simulink model "main"  (R2025b)
settings: Solver=FixedStepDiscrete  StartTime=0.0  StopTime=Inf  RelTol=1e-3  EnableMultiTasking=on
PreLoadFcn:
  | RTWConfigurationCB('preloadfcn', bdroot);
model workspace (MAT data in the model file):
  fault_count = 0
  fz_values = [0 50 100 150 200 250 300 350 400 450 500 550 ... (43 elements, 1x43)]
  k_opt_lut = [0 0 0 0 0 0 0 0 0 0 0 0 ... (4386 elements, 51x2x43)]
  mu_opt_lut = [0 0 0 0 0 0 0 0 0 0 0 0 ... (4386 elements, 51x2x43)]
undefined symbols (not defined in the file or in its folder): bit, Call, Function, ocv_lut, slope_lut, soc_lut
libraries: c2837xDlib x34, c280xlib x20, canmsglib x18, c2802xlib x12, simulink x9, slpidlib x3
(part 4 of 5)

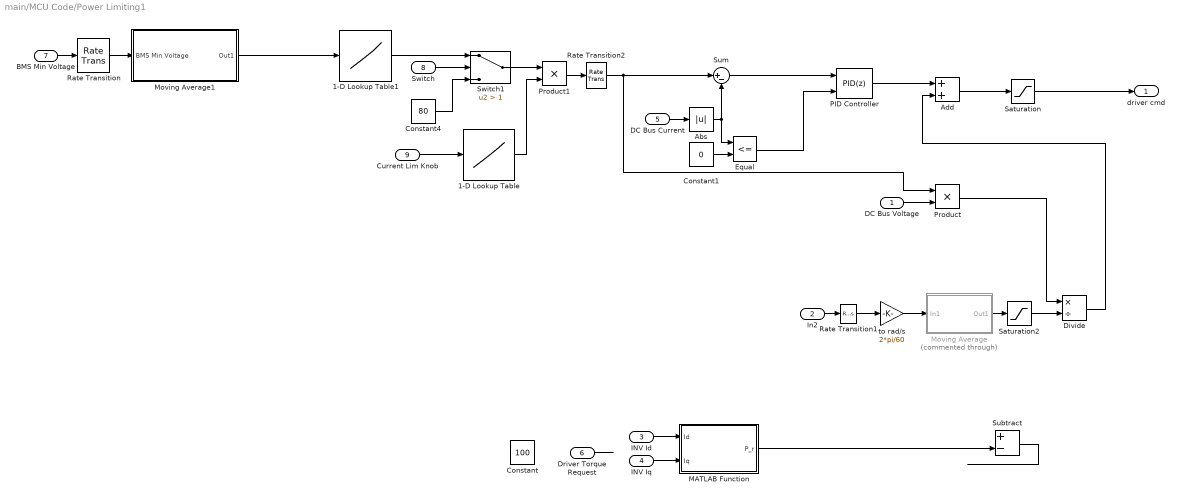
== system main/MCU Code/Power Limiting1 ==
  DC Bus Voltage : Inport
  In2 : Inport  Port=2
  INV Id : Inport  Port=3
  INV Iq : Inport  Port=4
  DC Bus Current : Inport  Port=5
  Driver Torque Request : Inport  Port=6
  BMS Min Voltage : Inport  Port=7
  Switch : Inport  Port=8
  Current Lim Knob : Inport  Port=9
  1-D Lookup Table : Lookup_n-D  NumberOfTableDimensions=1  BreakpointsForDimension1=[1 10]  Table=[0.1 1]  ExtrapMethod=Clip  UseLastTableValue=on  InternalRulePriority=Speed  RndMeth=Simplest
  1-D Lookup Table1 : Lookup_n-D  NumberOfTableDimensions=1  BreakpointsForDimension1=[3.4 4]  Table=[40 80]  ExtrapMethod=Clip  UseLastTableValue=on  InternalRulePriority=Speed  RndMeth=Simplest
  Abs : Abs  SaturateOnIntegerOverflow=off
  Add : Sum
  Constant : Constant  Value=100
  Constant1 : Constant  Value=0
  Constant4 : Constant  Value=80
  Divide : Product  Inputs=*/
  Equal : RelationalOperator  Operator=<=  OutDataTypeStr=boolean  RndMeth=Simplest  InputSameDT=off
  MATLAB Function : MATLAB Function  TreatAsAtomicUnit=on
  Moving Average : Subsystem  Commented=through
  Moving Average1 : Subsystem
  PID Controller : slpidlib/PID Controller  Controller=PID  Form=Parallel  TimeDomain=Discrete-time  UseExternalTs=off  SampleTime=-1  IntegratorMethod=Forward Euler  FilterMethod=Forward Euler  ControllerParametersSource=internal  P=0.45  I=10.8  UseKiTs=off  D=0  UseExternalDerivativeSource=off  N=100  UseFilter=on  TunerSelectOption=Transfer Function Based (PID Tuner App)  InitialConditionSource=internal  InitialConditionForIntegrator=0  InitialConditionForFilter=0  DifferentiatorICPrevScaledInput=0  ExternalReset=level  TrackingMode=off  Kt=1  LimitOutput=on  SatLimitsSource=internal  UpperSaturationLimit=inf  LowerSaturationLimit=-1000  LinearizeAsGain=off  AntiWindupMode=clamping  Kb=1  LimitIntegrator=on  UpperIntegratorSaturationLimit=0  LowerIntegratorSaturationLimit=-1000  POutMin=[]  POutMax=[]  IOutMin=[]  IOutMax=[]  DOutMin=[]  DOutMax=[]  NOutMin=[]  NOutMax=[]  SumOutMin=[]  SumOutMax=[]  SaturationOutMin=[]  SaturationOutMax=[]  PParamMin=[]  PParamMax=[]  IParamMin=[]  IParamMax=[]  DParamMin=[]  DParamMax=[]  NParamMin=[]  NParamMax=[]  KbParamMin=[]  KbParamMax=[]  KtParamMin=[]  KtParamMax=[]  KbOutMin=[]  KbOutMax=[]  KtOutMin=[]  KtOutMax=[]  IntegratorOutMin=[]  IntegratorOutMax=[]  FilterOutMin=[]  FilterOutMax=[]  SumI1OutMin=[]  SumI1OutMax=[]  SumI2OutMin=[]  SumI2OutMax=[]  SumI3OutMin=[]  SumI3OutMax=[]  SumI4OutMin=[]  SumI4OutMax=[]  SumDOutMin=[]  SumDOutMax=[]  DifferentiatorOutMin=[]  DifferentiatorOutMax=[]  FilterDiffOutCoefMin=[]  FilterDiffOutCoefMax=[]  ReciprocalOutMin=[]  ReciprocalOutMax=[]  SumDenOutMin=[]  SumDenOutMax=[]  SumNumOutMin=[]  SumNumOutMax=[]  DivideOutMin=[]  DivideOutMax=[]  UdiffTsProdOutMin=[]  UdiffTsProdOutMax=[]  NTsProdOutMin=[]  NTsProdOutMax=[]  UintegralTsProdOutMin=[]  UintegralTsProdOutMax=[]  UngainTsProdOutMin=[]  UngainTsProdOutMax=[]  ClampingZeroOutDataTypeStr=Inherit: Inherit via back propagation  ClampingZeroOutMin=[]  ClampingZeroOutMax=[]  FilterDenConstantOutDataTypeStr=Inherit: Inherit via back propagation  FilterDenConstantOutMin=[]  FilterDenConstantOutMax=[]  PCopyOutDataTypeStr=Inherit: Inherit via back propagation  PCopyOutMin=[]  PCopyOutMax=[]  NCopyOutDataTypeStr=Inherit: Inherit via back propagation  NCopyOutMin=[]  NCopyOutMax=[]  IntegratorContinuousStateAttributes=''  IntegratorStateMustResolveToSignalObject=off  IntegratorRTWStateStorageClass=Auto  FilterContinuousStateAttributes=''  FilterStateMustResolveToSignalObject=off  FilterRTWStateStorageClass=Auto  ParallelPVariant=InternalParameters  IdealPVariant=Disabled  IVariant=InternalParameters  DVariant=InternalParameters  IntegratorVariant=Discrete  SatVariant=Enabled  AWVariant=DiscClampingParallel  PCopyVariant=Disabled  TRVariant=Disabled  FdbkBlocksVariant=Forward  IdealPFdbkVariant=Disabled  SatFdbkVariant=Disabled  DerivativeFilterVariant=ForwardEulerFilter  NVariant=InternalParameters  NCopyVariant=Disabled  FilterICVariant=InternalICsFilter  IntegratorICVariant=InternalICs  ExternalResetVariant=ExternalReset  TRSumVariant=Passthrough  SumFdbkVariant=Disabled  SumVariant=Sum_PID  TsampFilterVariant=InternalTs  TsampNgainVariant=Passthrough  TsampIntegralVariant=Disabled_SignalSpec  ExternalSaturationOutDataTypeStr=Inherit: Same as second input  DerivativeSourceVariant=ErrorSignal  PreIntVariant=InternalPreInt
  Product : Product
  Product1 : Product
  Rate Transition : RateTransition  InitialCondition=1/5
  Rate Transition1 : RateTransition  OutPortSampleTime=0.001
  Rate Transition2 : RateTransition  OutPortSampleTime=0.001
  Saturation : Saturate  UpperLimit=inf  LowerLimit=0
  Saturation2 : Saturate  UpperLimit=inf  LowerLimit=1
  Subtract : Sum  Inputs=+-
  Sum : Sum  Inputs=|+-
  Switch1 : Switch  Criteria=u2 > Threshold  Threshold=1  SaturateOnIntegerOverflow=off  InputSameDT=off
  to rad/s : Gain  Gain=2*pi/60
  driver cmd : Outport
  wires:
  to rad/s/1 -> Moving Average/1(In1)
  Moving Average/1(Out1) -> Saturation2/1
  Saturation2/1 -> Divide/2
  Product/1 -> Divide/1
  DC Bus Voltage/1 -> Product/2
  In2/1 -> Rate Transition1/1
  INV Id/1 -> MATLAB Function/1(Id)
  INV Iq/1 -> MATLAB Function/2(Iq)
  MATLAB Function/1(P_r) -> Subtract/2
  Subtract/1 -> ?
  DC Bus Current/1 -> Abs/1
  Sum/1 -> PID Controller/1
  PID Controller/1 -> Add/1
  Driver Torque Request/1 -> ?
  Add/1 -> Saturation/1
  Abs/1 -> Sum/2, Equal/1
  Equal/1 -> PID Controller/2
  Product1/1 -> Rate Transition2/1
  Saturation/1 -> driver cmd/1
  Divide/1 -> Add/2
  Constant1/1 -> Equal/2
  BMS Min Voltage/1 -> Rate Transition/1
  Rate Transition/1 -> Moving Average1/1(BMS Min Voltage)
  Constant4/1 -> Switch1/3
  1-D Lookup Table1/1 -> Switch1/1
  Moving Average1/1(Out1) -> 1-D Lookup Table1/1
  Current Lim Knob/1 -> 1-D Lookup Table/1
  Switch1/1 -> Product1/1
  Switch/1 -> Switch1/2
  1-D Lookup Table/1 -> Product1/2
  Rate Transition2/1 -> Product/1, Sum/1
  Rate Transition1/1 -> to rad/s/1

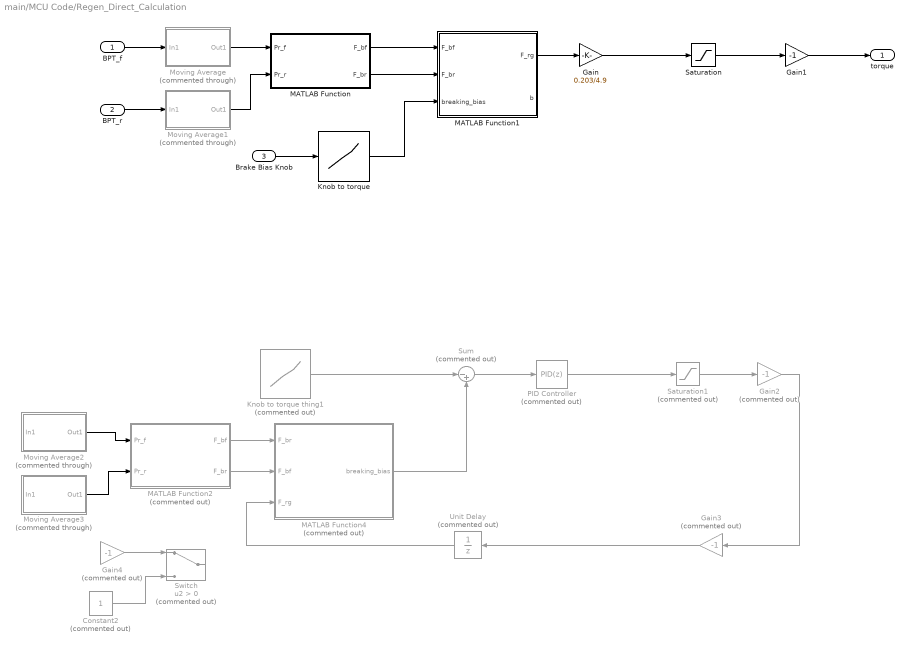
== system main/MCU Code/Regen_Direct_Calculation ==
  BPT_f : Inport
  BPT_r : Inport  Port=2
  Brake Bias Knob : Inport  Port=3
  Constant2 : Constant  Commented=on
  Gain : Gain  Gain=0.203/4.9
  Gain1 : Gain  Gain=-1
  Gain2 : Gain  Commented=on  Gain=-1
  Gain3 : Gain  Commented=on  Gain=-1
  Gain4 : Gain  Commented=on  Gain=-1
  Knob to torque : Lookup_n-D  NumberOfTableDimensions=1  BreakpointsForDimension1=[1 10]  Table=[0 1]  InternalRulePriority=Speed  RndMeth=Simplest
  Knob to torque thing1 : Lookup_n-D  Commented=on  NumberOfTableDimensions=1  BreakpointsForDimension1=[1 10]  Table=[0 1]  InternalRulePriority=Speed  RndMeth=Simplest
  MATLAB Function : MATLAB Function  TreatAsAtomicUnit=on
  MATLAB Function1 : MATLAB Function  TreatAsAtomicUnit=on
  MATLAB Function2 : MATLAB Function  Commented=on  TreatAsAtomicUnit=on
  MATLAB Function4 : MATLAB Function  Commented=on  TreatAsAtomicUnit=on
  Moving Average : Subsystem  Commented=through
  Moving Average1 : Subsystem  Commented=through
  Moving Average2 : Subsystem  Commented=through
  Moving Average3 : Subsystem  Commented=through
  PID Controller : slpidlib/PID Controller  Commented=on  Controller=PID  Form=Parallel  TimeDomain=Discrete-time  UseExternalTs=off  SampleTime=-1  IntegratorMethod=Forward Euler  FilterMethod=Forward Euler  ControllerParametersSource=internal  P=30  I=5000  UseKiTs=off  D=0  UseExternalDerivativeSource=off  N=100  UseFilter=on  TunerSelectOption=Transfer Function Based (PID Tuner App)  InitialConditionSource=internal  InitialConditionForIntegrator=0  InitialConditionForFilter=0  DifferentiatorICPrevScaledInput=0  ExternalReset=none  TrackingMode=off  Kt=1  LimitOutput=on  SatLimitsSource=internal  UpperSaturationLimit=inf  LowerSaturationLimit=-inf  LinearizeAsGain=on  AntiWindupMode=clamping  Kb=1  LimitIntegrator=off  UpperIntegratorSaturationLimit=inf  LowerIntegratorSaturationLimit=-inf  POutMin=[]  POutMax=[]  IOutMin=[]  IOutMax=[]  DOutMin=[]  DOutMax=[]  NOutMin=[]  NOutMax=[]  SumOutMin=[]  SumOutMax=[]  SaturationOutMin=[]  SaturationOutMax=[]  PParamMin=[]  PParamMax=[]  IParamMin=[]  IParamMax=[]  DParamMin=[]  DParamMax=[]  NParamMin=[]  NParamMax=[]  KbParamMin=[]  KbParamMax=[]  KtParamMin=[]  KtParamMax=[]  KbOutMin=[]  KbOutMax=[]  KtOutMin=[]  KtOutMax=[]  IntegratorOutMin=[]  IntegratorOutMax=[]  FilterOutMin=[]  FilterOutMax=[]  SumI1OutMin=[]  SumI1OutMax=[]  SumI2OutMin=[]  SumI2OutMax=[]  SumI3OutMin=[]  SumI3OutMax=[]  SumI4OutMin=[]  SumI4OutMax=[]  SumDOutMin=[]  SumDOutMax=[]  DifferentiatorOutMin=[]  DifferentiatorOutMax=[]  FilterDiffOutCoefMin=[]  FilterDiffOutCoefMax=[]  ReciprocalOutMin=[]  ReciprocalOutMax=[]  SumDenOutMin=[]  SumDenOutMax=[]  SumNumOutMin=[]  SumNumOutMax=[]  DivideOutMin=[]  DivideOutMax=[]  UdiffTsProdOutMin=[]  UdiffTsProdOutMax=[]  NTsProdOutMin=[]  NTsProdOutMax=[]  UintegralTsProdOutMin=[]  UintegralTsProdOutMax=[]  UngainTsProdOutMin=[]  UngainTsProdOutMax=[]  ClampingZeroOutDataTypeStr=Inherit: Inherit via back propagation  ClampingZeroOutMin=[]  ClampingZeroOutMax=[]  FilterDenConstantOutDataTypeStr=Inherit: Inherit via back propagation  FilterDenConstantOutMin=[]  FilterDenConstantOutMax=[]  PCopyOutDataTypeStr=Inherit: Inherit via back propagation  PCopyOutMin=[]  PCopyOutMax=[]  NCopyOutDataTypeStr=Inherit: Inherit via back propagation  NCopyOutMin=[]  NCopyOutMax=[]  IntegratorContinuousStateAttributes=''  IntegratorStateMustResolveToSignalObject=off  IntegratorRTWStateStorageClass=Auto  FilterContinuousStateAttributes=''  FilterStateMustResolveToSignalObject=off  FilterRTWStateStorageClass=Auto  ParallelPVariant=InternalParameters  IdealPVariant=Disabled  IVariant=InternalParameters  DVariant=InternalParameters  IntegratorVariant=Discrete  SatVariant=Enabled  AWVariant=DiscClampingParallel  PCopyVariant=Disabled  TRVariant=Disabled  FdbkBlocksVariant=Forward  IdealPFdbkVariant=Disabled  SatFdbkVariant=Disabled  DerivativeFilterVariant=ForwardEulerFilter  NVariant=InternalParameters  NCopyVariant=Disabled  FilterICVariant=InternalICsFilter  IntegratorICVariant=InternalICs  ExternalResetVariant=Disabled  TRSumVariant=Passthrough  SumFdbkVariant=Disabled  SumVariant=Sum_PID  TsampFilterVariant=InternalTs  TsampNgainVariant=Passthrough  TsampIntegralVariant=Disabled_SignalSpec  ExternalSaturationOutDataTypeStr=Inherit: Same as second input  DerivativeSourceVariant=ErrorSignal  PreIntVariant=InternalPreInt
  Saturation : Saturate  UpperLimit=100  LowerLimit=0
  Saturation1 : Saturate  Commented=on  UpperLimit=100  LowerLimit=0
  Sum : Sum  Commented=on  Inputs=|-+
  Switch : Switch  Commented=on  Criteria=u2 > Threshold  SaturateOnIntegerOverflow=off  InputSameDT=off
  Unit Delay : UnitDelay  Commented=on  SampleTime=-1  HasFrameUpgradeWarning=on
  torque : Outport
  wires:
  Gain1/1 -> torque/1
  Gain/1 -> Saturation/1
  Brake Bias Knob/1 -> Knob to torque/1
  BPT_f/1 -> Moving Average/1(In1)
  BPT_r/1 -> Moving Average1/1(In1)
  MATLAB Function/1(F_bf) -> MATLAB Function1/1(F_bf)
  MATLAB Function/2(F_br) -> MATLAB Function1/2(F_br)
  MATLAB Function1/1(F_rg) -> Gain/1
  Moving Average/1(Out1) -> MATLAB Function/1(Pr_f)
  Moving Average1/1(Out1) -> MATLAB Function/2(Pr_r)
  Knob to torque/1 -> MATLAB Function1/3(breaking_bias)
  ? -> Moving Average2/1(In1)
  Moving Average2/1(Out1) -> MATLAB Function2/1(Pr_f)
  Sum/1 -> PID Controller/1
  PID Controller/1 -> Saturation1/1
  MATLAB Function2/1(F_bf) -> MATLAB Function4/1(F_br)
  ? -> Moving Average3/1(In1)
  Saturation1/1 -> Gain2/1
  MATLAB Function4/1(breaking_bias) -> Sum/2
  Knob to torque thing1/1 -> Sum/1
  MATLAB Function2/2(F_br) -> MATLAB Function4/2(F_bf)
  Unit Delay/1 -> MATLAB Function4/3(F_rg)
  Moving Average3/1(Out1) -> MATLAB Function2/2(Pr_r)
  Gain3/1 -> Unit Delay/1
  Gain4/1 -> Switch/1
  ? -> Gain4/1
  Constant2/1 -> Switch/3
  ? -> Switch/2
  Saturation/1 -> Gain1/1
  Gain2/1 -> Gain3/1

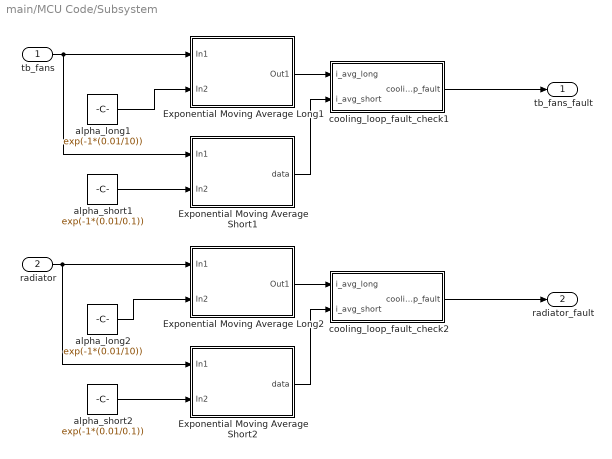
== system main/MCU Code/Subsystem ==
  tb_fans : Inport
  radiator : Inport  Port=2
  Exponential Moving Average Long1 : Subsystem
  Exponential Moving Average Long2 : Subsystem
  Exponential Moving Average Short1 : Subsystem
  Exponential Moving Average Short2 : Subsystem
  alpha_long1 : Constant  Value=exp(-1*(0.01/10))  VectorParams1D=off
  alpha_long2 : Constant  Value=exp(-1*(0.01/10))
  alpha_short1 : Constant  Value=exp(-1*(0.01/0.1))
  alpha_short2 : Constant  Value=exp(-1*(0.01/0.1))
  cooling_loop_fault_check1 : MATLAB Function  TreatAsAtomicUnit=on
  cooling_loop_fault_check2 : MATLAB Function  TreatAsAtomicUnit=on
  tb_fans_fault : Outport
  radiator_fault : Outport  Port=2
  wires:
  alpha_long1/1 -> Exponential Moving Average Long1/2(In2)
  Exponential Moving Average Short2/1(data) -> cooling_loop_fault_check2/2(i_avg_short)
  Exponential Moving Average Short1/1(data) -> cooling_loop_fault_check1/2(i_avg_short)
  Exponential Moving Average Long1/1(Out1) -> cooling_loop_fault_check1/1(i_avg_long)
  Exponential Moving Average Long2/1(Out1) -> cooling_loop_fault_check2/1(i_avg_long)
  alpha_long2/1 -> Exponential Moving Average Long2/2(In2)
  alpha_short1/1 -> Exponential Moving Average Short1/2(In2)
  alpha_short2/1 -> Exponential Moving Average Short2/2(In2)
  cooling_loop_fault_check1/1(cooling_loop_fault) -> tb_fans_fault/1
  cooling_loop_fault_check2/1(cooling_loop_fault) -> radiator_fault/1
  tb_fans/1 -> Exponential Moving Average Short1/1(In1), Exponential Moving Average Long1/1(In1)
  radiator/1 -> Exponential Moving Average Short2/1(In1), Exponential Moving Average Long2/1(In1)

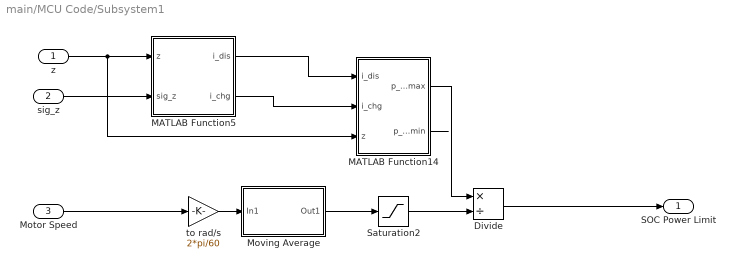
== system main/MCU Code/Subsystem1 ==
  z : Inport
  sig_z : Inport  Port=2
  Motor Speed : Inport  Port=3
  Divide : Product  Inputs=*/
  MATLAB Function14 : MATLAB Function  TreatAsAtomicUnit=on
  MATLAB Function5 : MATLAB Function  TreatAsAtomicUnit=on
  Moving Average : Subsystem
  Saturation2 : Saturate  UpperLimit=inf  LowerLimit=1
  to rad/s : Gain  Gain=2*pi/60
  SOC Power Limit : Outport
  wires:
  to rad/s/1 -> Moving Average/1(In1)
  MATLAB Function5/2(i_chg) -> MATLAB Function14/2(i_chg)
  Saturation2/1 -> Divide/2
  Motor Speed/1 -> to rad/s/1
  Moving Average/1(Out1) -> Saturation2/1
  MATLAB Function14/1(p_dis_max) -> Divide/1
  z/1 -> MATLAB Function5/1(z), MATLAB Function14/3(z)
  MATLAB Function5/1(i_dis) -> MATLAB Function14/1(i_dis)
  Divide/1 -> SOC Power Limit/1
  MATLAB Function14/2(p_chg_min) -> ?
  sig_z/1 -> MATLAB Function5/2(sig_z)

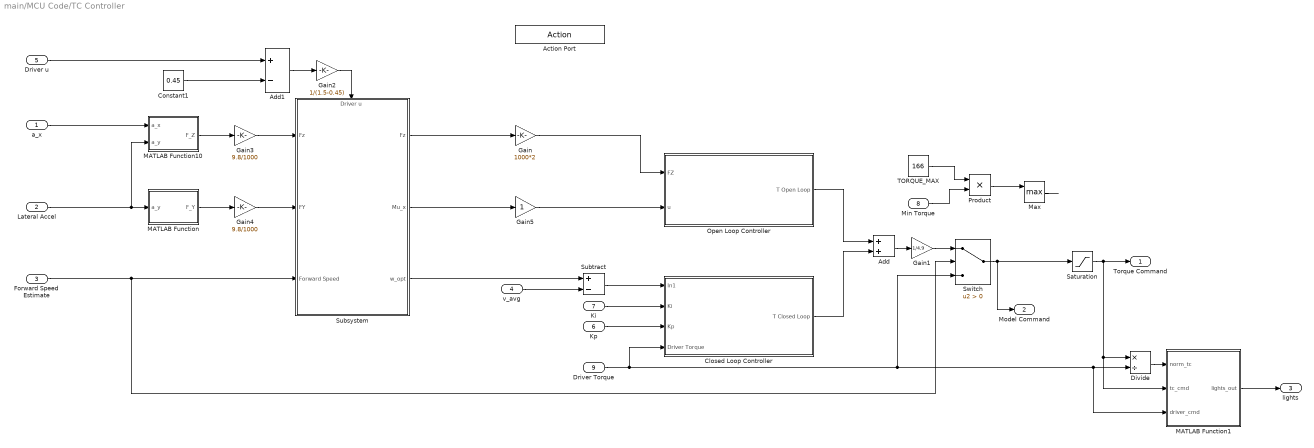
== system main/MCU Code/TC Controller ==
  a_x : Inport
  Lateral Accel : Inport  Port=2
  Forward Speed Estimate : Inport  Port=3
  v_avg : Inport  Port=4
  Driver u : Inport  Port=5
  Kp : Inport  Port=6
  Ki : Inport  Port=7
  Min Torque : Inport  Port=8
  Driver Torque : Inport  Port=9
  Action Port : ActionPort  ActionPortLabel=|
      | if(u1 == 1 | u1 == 3
      | )
  Add : Sum
  Add1 : Sum  Inputs=+-
  Closed Loop Controller : Subsystem
  Constant1 : Constant  Value=0.45
  Divide : Product  Inputs=*/
  Gain : Gain  Gain=1000*2
  Gain1 : Gain  Gain=1/4.9
  Gain2 : Gain  Gain=1/(1.5-0.45)
  Gain3 : Gain  Gain=9.8/1000
  Gain4 : Gain  Gain=9.8/1000
  Gain5 : Gain
  MATLAB Function : MATLAB Function  TreatAsAtomicUnit=on
  MATLAB Function1 : MATLAB Function  TreatAsAtomicUnit=on
  MATLAB Function10 : MATLAB Function  TreatAsAtomicUnit=on
  Max : MinMax  Function=max  Inputs=2
  Open Loop Controller : Subsystem
  Product : Product
  Saturation : Saturate  UpperLimit=166  LowerLimit=0
  Subsystem : Subsystem
      settings: PortSchema="{\"entries\":[{\"content\":{\"sides\":[{\"content\":{\"connectorIds\":[\"In1\",\"In2\",\"In3\"]},\"type\":\"ConnectorPlacement.EquallySpacedRectSide\",\"uuid\":\"52cb1509-e05e-4bae-af08-b3cbe80ce8d7\"},{\"content\":{\"connectorIds\":[\"Out1\",\"Out2\",\"Out3\"],\"side\":\"RIGHT\"},\"type\":\"ConnectorPlacement.EquallySpacedRectSide\",\"uuid\":\"5c1b6c4d-f36b-4262-971d-310d950de965\"},{\"content\":{\"connectorIds\":[\"In4\"],\"side\":\"TOP\"},\"type\":\"ConnectorPlacement.EquallySpacedRectSide\",\"uuid\":\"90df2961-afb4-4b60-bc78-aaa8af520e7a\"}]},\"type\":\"ConnectorPlacement.EquallySpacedConnector\",\"uuid\":\"073ed346-9857-4a79-b76f-e1da7d32971a\"}],\"packageUris\":[\"http://schema.mathworks.com/mf0/Connector/R2020b\"],\"version\":\"1.0\"}"
  Subtract : Sum  Inputs=+-
  Switch : Switch  Criteria=u2 > Threshold  SaturateOnIntegerOverflow=off  InputSameDT=off
  TORQUE_MAX : Constant  Value=166
  Torque Command : Outport
  Model Command : Outport  Port=2
  lights : Outport  Port=3
  wires:
  Gain1/1 -> Switch/1
  MATLAB Function10/1(F_Z) -> Gain3/1
  Open Loop Controller/1(T Open Loop) -> Add/1
  Closed Loop Controller/1(T Closed Loop) -> Add/2
  Add/1 -> Gain1/1
  v_avg/1 -> Subtract/2
  Kp/1 -> Closed Loop Controller/3(Kp)
  Forward Speed Estimate/1 -> Subsystem/3(Forward Speed), Switch/2
  Ki/1 -> Closed Loop Controller/2(Ki)
  Switch/1 -> Saturation/1, Model Command/1
  TORQUE_MAX/1 -> Product/1
  Min Torque/1 -> Product/2
  Lateral Accel/1 -> MATLAB Function10/2(a_y), MATLAB Function/1(a_y)
  Driver u/1 -> Add1/1
  Constant1/1 -> Add1/2
  Add1/1 -> Gain2/1
  Gain2/1 -> Subsystem/4(Driver u)
  Subsystem/3(w_opt) -> Subtract/1
  Subsystem/1(Fz) -> Gain/1
  Subsystem/2(Mu_x) -> Gain5/1
  Gain4/1 -> Subsystem/2(FY)
  MATLAB Function/1(F_Y) -> Gain4/1
  Gain3/1 -> Subsystem/1("Fz ")
  a_x/1 -> MATLAB Function10/1(a_x)
  Gain/1 -> Open Loop Controller/1(FZ)
  Gain5/1 -> Open Loop Controller/2(u)
  Subtract/1 -> Closed Loop Controller/1(In1)
  Saturation/1 -> Divide/1, MATLAB Function1/2(tc_cmd), Torque Command/1
  Max/1 -> ?
  Product/1 -> Max/1
  Driver Torque/1 -> Closed Loop Controller/4(Driver Torque), Switch/3, MATLAB Function1/3(driver_cmd), Divide/2
  Divide/1 -> MATLAB Function1/1(norm_tc)
  MATLAB Function1/1(lights_out) -> lights/1

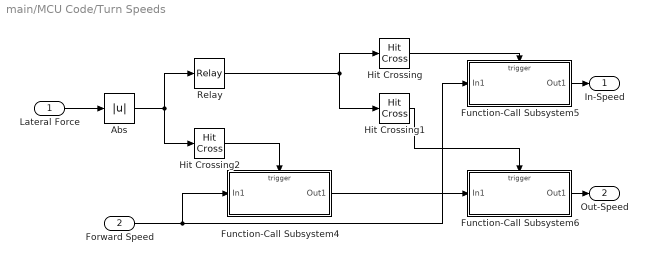
== system main/MCU Code/Turn Speeds ==
  Lateral Force : Inport
  Forward Speed : Inport  Port=2
  Abs : Abs  SaturateOnIntegerOverflow=off
  Function-Call Subsystem4 : Subsystem  TreatAsAtomicUnit=on
  Function-Call Subsystem5 : Subsystem  TreatAsAtomicUnit=on
  Function-Call Subsystem6 : Subsystem  TreatAsAtomicUnit=on
  Hit Crossing : HitCross  HitCrossingOffset=0.5  HitCrossingDirection=rising  HitCrossingOutputType=Function-Call
  Hit Crossing1 : HitCross  HitCrossingOffset=0.5  HitCrossingDirection=falling  HitCrossingOutputType=Function-Call
  Hit Crossing2 : HitCross  HitCrossingOffset=1  HitCrossingOutputType=Function-Call
  Relay : Relay  OnSwitchValue=1  OffSwitchValue=0.5
  In-Speed : Outport
  Out-Speed : Outport  Port=2
  wires:
  Forward Speed/1 -> Function-Call Subsystem4/1(In1), Function-Call Subsystem5/1(In1)
  Hit Crossing2/1 -> Function-Call Subsystem4/Trigger
  Function-Call Subsystem4/1(Out1) -> Function-Call Subsystem6/1(In1)
  Relay/1 -> Hit Crossing1/1, Hit Crossing/1
  Hit Crossing1/1 -> Function-Call Subsystem6/Trigger
  Hit Crossing/1 -> Function-Call Subsystem5/Trigger
  Function-Call Subsystem5/1(Out1) -> In-Speed/1
  Lateral Force/1 -> Abs/1
  Function-Call Subsystem6/1(Out1) -> Out-Speed/1
  Abs/1 -> Relay/1, Hit Crossing2/1

== system main/Subsystem/Subsystem3 ==
  In1 : Inport
  In2 : Inport  Port=2
  Forward Speed Estimate : Inport  Port=3
  In4 : Inport  Port=4
  Enable : EnablePort

== system main/MCU Code/Kalman Filter/Kalman1 ==
  Accel : Inport
  Speed F : Inport  Port=2
  Accel update : Inport  Port=3
  Velocity Update : Inport  Port=4
  Time : Inport  Port=5
  MATLAB System : MATLABSystem  System=Kalman_Filter_Mod  qgain=1  SimulateUsing=Code generation
      mask Type: Kalman_Filter_Mod
  Forward Speed : Outport
  Accel Estimate : Outport  Port=2
  Error Covariance : Outport  Port=3
  wires:
  Speed F/1 -> MATLAB System/2
  Accel/1 -> MATLAB System/1
  MATLAB System/1 -> Forward Speed/1
  Accel update/1 -> MATLAB System/3
  Velocity Update/1 -> MATLAB System/4
  Time/1 -> MATLAB System/5
  MATLAB System/2 -> Accel Estimate/1
  MATLAB System/3 -> Error Covariance/1

== system main/MCU Code/Kalman Filter/Sensor Driver 1 ==
  In1 : Inport
  Circumference : Gain  Gain=2*pi*0.203
  Gain : Gain  Gain=3.6
  Inverse Teeth : Gain  Gain=1/21
  " " : Outport
  wires:
  In1/1 -> Gain/1
  Gain/1 -> Circumference/1
  Circumference/1 -> Inverse Teeth/1
  Inverse Teeth/1 -> " "/1

== system main/MCU Code/Kalman Filter/Sensor Driver 2 ==
  In1 : Inport
  Circumference : Gain  Gain=2*pi*0.203
  Gain : Gain  Gain=3.6
  Inverse Teeth : Gain  Gain=1/21
  " " : Outport
  wires:
  Circumference/1 -> Inverse Teeth/1
  Inverse Teeth/1 -> " "/1
  In1/1 -> Gain/1
  Gain/1 -> Circumference/1

== system main/MCU Code/Kalman Filter/Sensor Driver 3 ==
  In1 : Inport
  Circumference : Gain  Gain=2*pi*0.203
  Gain : Gain  Gain=3.6
  Inverse Teeth : Gain  Gain=1/21
  RL : Outport
  wires:
  Circumference/1 -> Inverse Teeth/1
  Inverse Teeth/1 -> RL/1
  In1/1 -> Gain/1
  Gain/1 -> Circumference/1

== system main/MCU Code/Kalman Filter/Sensor Driver 4 ==
  In1 : Inport
  Circumference : Gain  Gain=2*pi*0.203
  Gain : Gain  Gain=3.6
  Inverse Teeth : Gain  Gain=1/21
  RR : Outport
  wires:
  Circumference/1 -> Inverse Teeth/1
  Inverse Teeth/1 -> RR/1
  In1/1 -> Gain/1
  Gain/1 -> Circumference/1

== system main/MCU Code/Kalman Filter/Slip Ratio Calculation1 ==
  RR : Inport
  Forward Speed : Inport  Port=2
  MATLAB Function : MATLAB Function  TreatAsAtomicUnit=on
  Slip Ratio : Outport
  wires:
  Forward Speed/1 -> MATLAB Function/1(fwd_speed)
  RR/1 -> MATLAB Function/2(v_rear)
  MATLAB Function/1(y) -> Slip Ratio/1

== system main/MCU Code/Power Limiting/Moving Average ==
  In1 : Inport
  Product1 : Product  Inputs=*/
  Saturation : Saturate  UpperLimit=inf  LowerLimit=1
  Sum of Elements : Sum  Inputs=+
  Tapped Delay : simulink/Discrete/Tapped Delay  vinit=0.0  samptime=-1  NumDelays=10  DelayOrder=Oldest  includeCurrent=on
  Width : Width
  Out1 : Outport
  wires:
  Tapped Delay/1 -> Width/1, Sum of Elements/1
  Sum of Elements/1 -> Product1/1
  Product1/1 -> Out1/1
  In1/1 -> Tapped Delay/1
  Width/1 -> Saturation/1
  Saturation/1 -> Product1/2

== system main/MCU Code/Power Limiting1/Moving Average ==
  In1 : Inport
  Product1 : Product  Inputs=*/
  Saturation : Saturate  UpperLimit=inf  LowerLimit=1
  Sum of Elements : Sum  Inputs=+
  Tapped Delay : simulink/Discrete/Tapped Delay  vinit=0.0  samptime=-1  NumDelays=10  DelayOrder=Oldest  includeCurrent=on
  Width : Width
  Out1 : Outport
  wires:
  Tapped Delay/1 -> Width/1, Sum of Elements/1
  Sum of Elements/1 -> Product1/1
  Product1/1 -> Out1/1
  In1/1 -> Tapped Delay/1
  Width/1 -> Saturation/1
  Saturation/1 -> Product1/2

== system main/MCU Code/Power Limiting1/Moving Average1 ==
  BMS Min Voltage : Inport
  Product1 : Product  Inputs=*/
  Saturation : Saturate  UpperLimit=inf  LowerLimit=1
  Sum of Elements : Sum  Inputs=+
  Tapped Delay : simulink/Discrete/Tapped Delay  vinit=0.0  samptime=-1  NumDelays=50  DelayOrder=Oldest  includeCurrent=on
  Width : Width
  Out1 : Outport
  wires:
  Tapped Delay/1 -> Width/1, Sum of Elements/1
  Sum of Elements/1 -> Product1/1
  Product1/1 -> Out1/1
  BMS Min Voltage/1 -> Tapped Delay/1
  Width/1 -> Saturation/1
  Saturation/1 -> Product1/2

== system main/MCU Code/Regen_Direct_Calculation/Moving Average ==
  In1 : Inport
  Product1 : Product  Inputs=*/
  Saturation : Saturate  UpperLimit=inf  LowerLimit=1
  Sum of Elements : Sum  Inputs=+
  Tapped Delay : simulink/Discrete/Tapped Delay  vinit=0.0  samptime=-1  NumDelays=10  DelayOrder=Oldest  includeCurrent=on
  Width : Width
  Out1 : Outport
  wires:
  Tapped Delay/1 -> Width/1, Sum of Elements/1
  Sum of Elements/1 -> Product1/1
  Product1/1 -> Out1/1
  In1/1 -> Tapped Delay/1
  Width/1 -> Saturation/1
  Saturation/1 -> Product1/2

== system main/MCU Code/Regen_Direct_Calculation/Moving Average1 ==
  In1 : Inport
  Product1 : Product  Inputs=*/
  Saturation : Saturate  UpperLimit=inf  LowerLimit=1
  Sum of Elements : Sum  Inputs=+
  Tapped Delay : simulink/Discrete/Tapped Delay  vinit=0.0  samptime=-1  NumDelays=10  DelayOrder=Oldest  includeCurrent=on
  Width : Width
  Out1 : Outport
  wires:
  Tapped Delay/1 -> Width/1, Sum of Elements/1
  Sum of Elements/1 -> Product1/1
  Product1/1 -> Out1/1
  In1/1 -> Tapped Delay/1
  Width/1 -> Saturation/1
  Saturation/1 -> Product1/2

== system main/MCU Code/Regen_Direct_Calculation/Moving Average2 ==
  In1 : Inport
  Product1 : Product  Inputs=*/
  Saturation : Saturate  UpperLimit=inf  LowerLimit=1
  Sum of Elements : Sum  Inputs=+
  Tapped Delay : simulink/Discrete/Tapped Delay  vinit=0.0  samptime=-1  NumDelays=10  DelayOrder=Oldest  includeCurrent=on
  Width : Width
  Out1 : Outport
  wires:
  Tapped Delay/1 -> Width/1, Sum of Elements/1
  Sum of Elements/1 -> Product1/1
  Product1/1 -> Out1/1
  In1/1 -> Tapped Delay/1
  Width/1 -> Saturation/1
  Saturation/1 -> Product1/2

== system main/MCU Code/Regen_Direct_Calculation/Moving Average3 ==
  In1 : Inport
  Product1 : Product  Inputs=*/
  Saturation : Saturate  UpperLimit=inf  LowerLimit=1
  Sum of Elements : Sum  Inputs=+
  Tapped Delay : simulink/Discrete/Tapped Delay  vinit=0.0  samptime=-1  NumDelays=10  DelayOrder=Oldest  includeCurrent=on
  Width : Width
  Out1 : Outport
  wires:
  Tapped Delay/1 -> Width/1, Sum of Elements/1
  Sum of Elements/1 -> Product1/1
  Product1/1 -> Out1/1
  In1/1 -> Tapped Delay/1
  Width/1 -> Saturation/1
  Saturation/1 -> Product1/2

== system main/MCU Code/Subsystem/Exponential Moving Average Long1 ==
  In1 : Inport
  In2 : Inport  Port=2
  Constant4 : Constant
  Delay One Step : Delay  DelayLength=1
  Product : Product
  Product1 : Product
  Subtract : Sum  Inputs=+-
  Sum : Sum  Inputs=|++
  Out1 : Outport
  wires:
  In2/1 -> Subtract/2, Product1/2
  Product1/1 -> Sum/1
  Subtract/1 -> Product/2
  Sum/1 -> Out1/1, Delay One Step/1
  Constant4/1 -> Subtract/1
  Product/1 -> Sum/2
  Delay One Step/1 -> Product/1
  In1/1 -> Product1/1

== system main/MCU Code/Subsystem/Exponential Moving Average Long2 ==
  In1 : Inport
  In2 : Inport  Port=2
  Constant4 : Constant
  Delay One Step : Delay  DelayLength=1
  Product : Product
  Product1 : Product
  Subtract : Sum  Inputs=+-
  Sum : Sum  Inputs=|++
  Out1 : Outport
  wires:
  In2/1 -> Subtract/2, Product1/2
  Product1/1 -> Sum/1
  Subtract/1 -> Product/2
  Sum/1 -> Out1/1, Delay One Step/1
  Constant4/1 -> Subtract/1
  Product/1 -> Sum/2
  Delay One Step/1 -> Product/1
  In1/1 -> Product1/1

== system main/MCU Code/Subsystem/Exponential Moving Average Short1 ==
  In1 : Inport
  In2 : Inport  Port=2
  Constant4 : Constant
  Delay One Step : Delay  DelayLength=1
  Product : Product
  Product1 : Product
  Subtract : Sum  Inputs=+-
  Sum : Sum  Inputs=|++
  data : Outport
  wires:
  In2/1 -> Subtract/2, Product1/2
  Product1/1 -> Sum/1
  Subtract/1 -> Product/2
  Sum/1 -> data/1, Delay One Step/1
  Constant4/1 -> Subtract/1
  Product/1 -> Sum/2
  Delay One Step/1 -> Product/1
  In1/1 -> Product1/1

== system main/MCU Code/Subsystem/Exponential Moving Average Short2 ==
  In1 : Inport
  In2 : Inport  Port=2
  Constant4 : Constant
  Delay One Step : Delay  DelayLength=1
  Product : Product
  Product1 : Product
  Subtract : Sum  Inputs=+-
  Sum : Sum  Inputs=|++
  data : Outport
  wires:
  In2/1 -> Subtract/2, Product1/2
  Product1/1 -> Sum/1
  Subtract/1 -> Product/2
  Sum/1 -> data/1, Delay One Step/1
  Constant4/1 -> Subtract/1
  Product/1 -> Sum/2
  Delay One Step/1 -> Product/1
  In1/1 -> Product1/1

== system main/MCU Code/Subsystem1/Moving Average ==
  In1 : Inport
  Product1 : Product  Inputs=*/
  Saturation : Saturate  UpperLimit=inf  LowerLimit=1
  Sum of Elements : Sum  Inputs=+
  Tapped Delay : simulink/Discrete/Tapped Delay  vinit=0.0  samptime=-1  NumDelays=10  DelayOrder=Oldest  includeCurrent=on
  Width : Width
  Out1 : Outport
  wires:
  Tapped Delay/1 -> Width/1, Sum of Elements/1
  Sum of Elements/1 -> Product1/1
  Product1/1 -> Out1/1
  In1/1 -> Tapped Delay/1
  Width/1 -> Saturation/1
  Saturation/1 -> Product1/2

== system main/MCU Code/TC Controller/Closed Loop Controller ==
  In1 : Inport
  Ki : Inport  Port=2
  Kp : Inport  Port=3
  Driver Torque : Inport  Port=4
  Constant : Constant  Value=0
  Equal : RelationalOperator  Operator===  OutDataTypeStr=boolean  RndMeth=Simplest  InputSameDT=off
  PID Controller : slpidlib/PID Controller  Controller=PI  Form=Parallel  TimeDomain=Discrete-time  UseExternalTs=off  SampleTime=-1  IntegratorMethod=Forward Euler  FilterMethod=Forward Euler  ControllerParametersSource=external  P=100  I=10  UseKiTs=off  D=0  UseExternalDerivativeSource=off  N=100  UseFilter=on  TunerSelectOption=Transfer Function Based (PID Tuner App)  InitialConditionSource=internal  InitialConditionForIntegrator=0  InitialConditionForFilter=0  DifferentiatorICPrevScaledInput=0  ExternalReset=level  TrackingMode=off  Kt=1  LimitOutput=on  SatLimitsSource=internal  UpperSaturationLimit=166*4.9  LowerSaturationLimit=-166*4.9  LinearizeAsGain=on  AntiWindupMode=clamping  Kb=1  LimitIntegrator=on  UpperIntegratorSaturationLimit=166*4.9  LowerIntegratorSaturationLimit=-166*4.9  POutMin=[]  POutMax=[]  IOutMin=[]  IOutMax=[]  DOutMin=[]  DOutMax=[]  NOutMin=[]  NOutMax=[]  SumOutMin=[]  SumOutMax=[]  SaturationOutMin=[]  SaturationOutMax=[]  PParamMin=[]  PParamMax=[]  IParamMin=[]  IParamMax=[]  DParamMin=[]  DParamMax=[]  NParamMin=[]  NParamMax=[]  KbParamMin=[]  KbParamMax=[]  KtParamMin=[]  KtParamMax=[]  KbOutMin=[]  KbOutMax=[]  KtOutMin=[]  KtOutMax=[]  IntegratorOutMin=[]  IntegratorOutMax=[]  FilterOutMin=[]  FilterOutMax=[]  SumI1OutMin=[]  SumI1OutMax=[]  SumI2OutMin=[]  SumI2OutMax=[]  SumI3OutMin=[]  SumI3OutMax=[]  SumI4OutMin=[]  SumI4OutMax=[]  SumDOutMin=[]  SumDOutMax=[]  DifferentiatorOutMin=[]  DifferentiatorOutMax=[]  FilterDiffOutCoefMin=[]  FilterDiffOutCoefMax=[]  ReciprocalOutMin=[]  ReciprocalOutMax=[]  SumDenOutMin=[]  SumDenOutMax=[]  SumNumOutMin=[]  SumNumOutMax=[]  DivideOutMin=[]  DivideOutMax=[]  UdiffTsProdOutMin=[]  UdiffTsProdOutMax=[]  NTsProdOutMin=[]  NTsProdOutMax=[]  UintegralTsProdOutMin=[]  UintegralTsProdOutMax=[]  UngainTsProdOutMin=[]  UngainTsProdOutMax=[]  ClampingZeroOutDataTypeStr=Inherit: Inherit via back propagation  ClampingZeroOutMin=[]  ClampingZeroOutMax=[]  FilterDenConstantOutDataTypeStr=Inherit: Inherit via back propagation  FilterDenConstantOutMin=[]  FilterDenConstantOutMax=[]  PCopyOutDataTypeStr=Inherit: Inherit via back propagation  PCopyOutMin=[]  PCopyOutMax=[]  NCopyOutDataTypeStr=Inherit: Inherit via back propagation  NCopyOutMin=[]  NCopyOutMax=[]  IntegratorContinuousStateAttributes=''  IntegratorStateMustResolveToSignalObject=off  IntegratorRTWStateStorageClass=Auto  FilterContinuousStateAttributes=''  FilterStateMustResolveToSignalObject=off  FilterRTWStateStorageClass=Auto  ParallelPVariant=ExternalParameters  IdealPVariant=Disabled  IVariant=ExternalParameters  DVariant=Disabled  IntegratorVariant=Discrete  SatVariant=Enabled  AWVariant=DiscClampingParallel  PCopyVariant=Disabled  TRVariant=Disabled  FdbkBlocksVariant=Forward  IdealPFdbkVariant=Disabled  SatFdbkVariant=Disabled  DerivativeFilterVariant=Disabled  NVariant=Disabled  NCopyVariant=Disabled_SignalSpec  FilterICVariant=Disabled  IntegratorICVariant=InternalICs  ExternalResetVariant=ExternalReset  TRSumVariant=Passthrough  SumFdbkVariant=Disabled  SumVariant=Sum_PI  TsampFilterVariant=InternalTs  TsampNgainVariant=Passthrough  TsampIntegralVariant=Disabled_SignalSpec  ExternalSaturationOutDataTypeStr=Inherit: Same as second input  DerivativeSourceVariant=Disabled  PreIntVariant=InternalPreInt
  T Closed Loop : Outport
  wires:
  In1/1 -> PID Controller/1
  PID Controller/1 -> T Closed Loop/1
  Kp/1 -> PID Controller/2
  Ki/1 -> PID Controller/3
  Driver Torque/1 -> Equal/1
  Equal/1 -> PID Controller/4
  Constant/1 -> Equal/2

== system main/MCU Code/TC Controller/Open Loop Controller ==
  FZ : Inport
  u : Inport  Port=2
  Gain : Gain  Gain=0.203
  Product : Product
  T Open Loop : Outport
  wires:
  FZ/1 -> Product/1
  u/1 -> Product/2
  Gain/1 -> T Open Loop/1
  Product/1 -> Gain/1

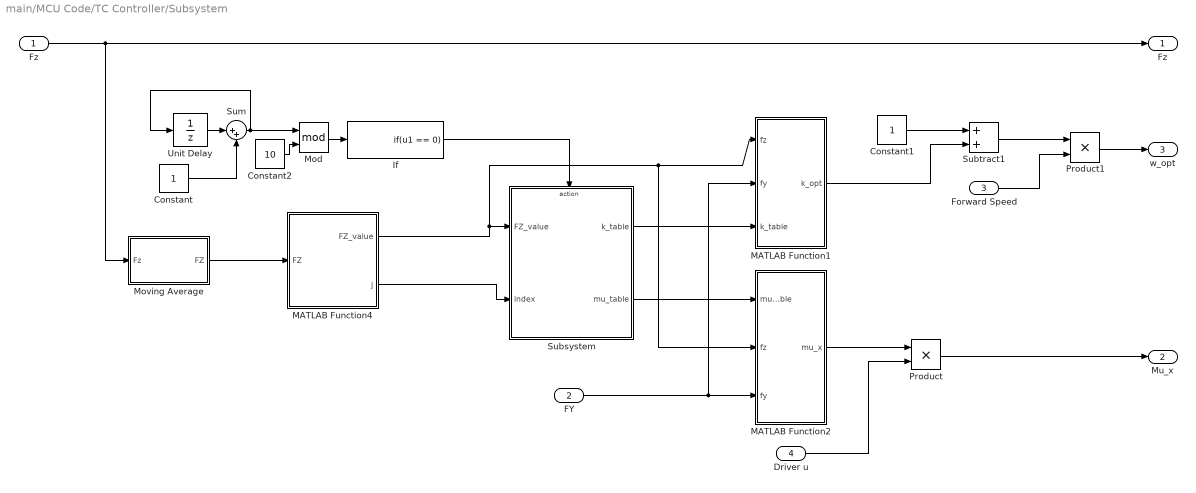
== system main/MCU Code/TC Controller/Subsystem ==
  "Fz " : Inport
  FY : Inport  Port=2
  Forward Speed : Inport  Port=3
  Driver u : Inport  Port=4
  Constant : Constant
  Constant1 : Constant
  Constant2 : Constant  Value=10
  If : If  IfExpression=u1 == 0  ShowElse=off  ZeroCross=off
  MATLAB Function1 : MATLAB Function  TreatAsAtomicUnit=on
  MATLAB Function2 : MATLAB Function  TreatAsAtomicUnit=on
  MATLAB Function4 : MATLAB Function  TreatAsAtomicUnit=on
  Mod : Math  Operator=mod
  Moving Average : Subsystem
  Product : Product
  Product1 : Product
  Subsystem : Subsystem
  Subtract1 : Sum
  Sum : Sum  Inputs=|++
  Unit Delay : UnitDelay  SampleTime=-1  HasFrameUpgradeWarning=on
  Fz : Outport
  Mu_x : Outport  Port=2
  w_opt : Outport  Port=3
  wires:
  Product1/1 -> w_opt/1
  Forward Speed/1 -> Product1/2
  "Fz "/1 -> Fz/1, Moving Average/1("Fz ")
  Product/1 -> Mu_x/1
  Constant1/1 -> Subtract1/1
  FY/1 -> MATLAB Function1/2(fy), MATLAB Function2/3(fy)
  Subtract1/1 -> Product1/1
  MATLAB Function1/1(k_opt) -> Subtract1/2
  Moving Average/1(FZ) -> MATLAB Function4/1(FZ)
  MATLAB Function4/1(FZ_value) -> MATLAB Function2/2(fz), MATLAB Function1/1(fz), Subsystem/1(FZ_value)
  MATLAB Function4/2(j) -> Subsystem/2(index)
  Sum/1 -> Unit Delay/1, Mod/1
  Unit Delay/1 -> Sum/1
  Constant2/1 -> Mod/2
  Constant/1 -> Sum/2
  Mod/1 -> If/1
  If/1 -> Subsystem/Action
  Subsystem/1(k_table) -> MATLAB Function1/3(k_table)
  Subsystem/2(mu_table) -> MATLAB Function2/1(mu_table)
  MATLAB Function2/1(mu_x) -> Product/1
  Driver u/1 -> Product/2

== system main/MCU Code/Turn Speeds/Function-Call Subsystem4 ==
  In1 : Inport
  function : TriggerPort  TriggerType=function-call  VariantControl=(inherit)
  Out1 : Outport
  wires:
  In1/1 -> Out1/1

== system main/MCU Code/Turn Speeds/Function-Call Subsystem5 ==
  In1 : Inport
  function : TriggerPort  TriggerType=function-call  VariantControl=(inherit)
  Out1 : Outport
  wires:
  In1/1 -> Out1/1

== system main/MCU Code/Turn Speeds/Function-Call Subsystem6 ==
  In1 : Inport
  function : TriggerPort  TriggerType=function-call  VariantControl=(inherit)
  Out1 : Outport
  wires:
  In1/1 -> Out1/1

== system main/MCU Code/TC Controller/Subsystem/Moving Average ==
  "Fz " : Inport
  Product1 : Product  Inputs=*/
  Saturation : Saturate  UpperLimit=inf  LowerLimit=1
  Sum of Elements : Sum  Inputs=+
  Tapped Delay : simulink/Discrete/Tapped Delay  vinit=0.0  samptime=-1  NumDelays=10  DelayOrder=Oldest  includeCurrent=on
  Width : Width
  FZ : Outport
  wires:
  Tapped Delay/1 -> Width/1, Sum of Elements/1
  Sum of Elements/1 -> Product1/1
  Product1/1 -> FZ/1
  "Fz "/1 -> Tapped Delay/1
  Width/1 -> Saturation/1
  Saturation/1 -> Product1/2

== system main/MCU Code/TC Controller/Subsystem/Subsystem ==
  FZ_value : Inport
  index : Inport  Port=2
  Action Port : ActionPort  ActionPortLabel=if(u1 == 0)
  MATLAB Function : MATLAB Function  TreatAsAtomicUnit=on
  k_table : Outport
  mu_table : Outport  Port=2
  wires:
  FZ_value/1 -> MATLAB Function/1(FZ_value)
  index/1 -> MATLAB Function/2(index)
  MATLAB Function/1(k_table) -> k_table/1
  MATLAB Function/2(mu_table) -> mu_table/1

== matlab function main/MCU Code/MATLAB Function11 ==
  data: bpt_f input; bpt_f_bar output; bpt_r input; bpt_r_bar output
function [bpt_f_bar,bpt_r_bar] = fcn(bpt_f,bpt_r)
bpt_f_bar = double((((single(bpt_f)/4095)*3.3*4)-0.5)*25);
bpt_r_bar = double((((single(bpt_r)/4095)*3.3*4)-0.5)*25);

%hi ben i hope u find this

== matlab function main/MCU Code/MATLAB Function ==
  data: ts input; ts_state output; length input; time_out output
function [ts_state, time_out] = fcn(ts, length)

% if timeout
%     out = -1; % timeout in TS state CAN signal
persistent timeout;
if isempty(timeout)
    timeout = 0;
end

if length == 0
    timeout = timeout + 1;
else
    timeout = 0;
end

if timeout > 200
    time_out = 1;
else
    time_out = 0;
end

ts_state = ts;

== stateflow chart main/MCU Code/Chart ==
  state State6_Motor_Disabled
    state=6;
    ready_led = 0;
    buzzer = 0;
    inverter_en = 0;
    dc_dc = 1;
    driving = 0;
  state State1_TS_NotReady
    state=1;
    ready_led = 0;
    buzzer = 0;
    inverter_en = 0;
    dc_dc = 0;
    driving = 0;
  state State7_Comms_Timeout
    state = 7;
    ready_led = 0;
    buzzer = 0;
    inverter_en = 0;
    dc_dc = 1;
    driving = 0;
  state State5_Ready_to_Drive
    state=5;
    ready_led = 0;
    buzzer = 0;
    inverter_en = 1;
    dc_dc = 1;
    driving = 1;
  state State8_E_Fuse
    state = 8;
    ready_led = 0;
    buzzer = 0;
    inverter_en = 0;
    dc_dc = 1;
    driving = 0;
  state State4_Enabling
    state=4;
    ready_led = 0;
    buzzer = 0;
    inverter_en = 1;
    dc_dc = 1;
    driving = 0;
  state State3_Buzzing
    state=3;
    ready_led = 0;
    buzzer = 1;
    inverter_en = 0;
    dc_dc = 1;
    driving = 0;
  state State2_TS_Ready
    state=2;
    ready_led = 1;
    buzzer = 0;
    inverter_en = 0;
    dc_dc = 0;
    driving = 0;
  State3_Buzzing -> State1_TS_NotReady [order 2] : [TS_state ~= 5 | SDC_Sig]
  State5_Ready_to_Drive -> State1_TS_NotReady [order 2] : [TS_state ~= 5 | SDC_Sig]
  State6_Motor_Disabled -> State1_TS_NotReady [order 1] : [TS_state ~= 5 | SDC_Sig]
  (default) -> State1_TS_NotReady
  State4_Enabling -> State6_Motor_Disabled [order 2] : [any(Pedal_Fault)]
  State6_Motor_Disabled -> State4_Enabling [order 2] : [~any(Pedal_Fault)]
  State5_Ready_to_Drive -> State6_Motor_Disabled [order 1] : [any(Pedal_Fault)]
  State7_Comms_Timeout -> State1_TS_NotReady [order 1] : [TS_state~=5 | SDC_Sig]
  State5_Ready_to_Drive -> State7_Comms_Timeout [order 4] : [ts_state_timeout]
  State2_TS_Ready -> State1_TS_NotReady [order 2] : [TS_state ~= 5 | SDC_Sig]
  State1_TS_NotReady -> State2_TS_Ready : [TS_state == 5 & ~SDC_Sig]
  State5_Ready_to_Drive -> State2_TS_Ready [order 3] : [INV_enable ~= 1]
  State5_Ready_to_Drive -> State8_E_Fuse [order 5] : [DC_Bus_Current > 200]
  State7_Comms_Timeout -> State2_TS_Ready [order 2] : [~ts_state_timeout]
  State8_E_Fuse -> State4_Enabling : after(5,sec)
  State4_Enabling -> State5_Ready_to_Drive [order 1] : [INV_enable==1]
  State3_Buzzing -> State4_Enabling [order 1] : after(3,sec)
  State2_TS_Ready -> State3_Buzzing [order 1] : [BPT==1&&RTD_Button==1]
  data: BPT input; RTD_Button input; Pedal_Fault input; ts_state_timeout input; SDC_Sig input; INV_enable input; TS_state input; state output; ready_led output; buzzer output; dc_dc output; inverter_en output; driving output; DC_Bus_Current input

== matlab function main/MCU Code/MATLAB Function5 ==
  data: brake_bias input; servo_pos output; mcu_control input
function servo_pos = fcn(brake_bias,mcu_control)

if(mcu_control == 2 | mcu_control == 3)
    servo_pos = 10;
else
    servo_pos = brake_bias; 
end

== matlab function main/MCU Code/MATLAB Function3 ==
  data: inv input; out output; length input
function out = fcn(inv, length)

% if timeout
%     out = -1; % timeout in TS state CAN signal
persistent timeout;
if isempty(timeout)
    timeout = 0;
end

if length == 0
    timeout = timeout + 1;
else
    timeout = 0;
end

if timeout > 4
    out = double(-1);
else
    out = double(inv);
end

== matlab function main/MCU Code/MATLAB Function4 ==
  data: sig input; APPS1_RANGE input; r_momentary input; percent output
function percent = map_apps1(sig, APPS1_RANGE, r_momentary)

DZ_BOT = .05; %rosnel changed to .05 was .1 
DZ_TOP = .05; 

APPS_BOTTOM = APPS1_RANGE(1) + DZ_BOT * (APPS1_RANGE(2) - APPS1_RANGE(1)) ;
APPS_TOP    = APPS1_RANGE(2) - DZ_TOP * (APPS1_RANGE(2) - APPS1_RANGE(1)) ;

if (sig > max(APPS1_RANGE)) || r_momentary(1) || r_momentary(2)
    percent = 0;
elseif (sig < min(APPS1_RANGE))
    percent = 1;
else
    percent = (double(sig) - APPS_BOTTOM) / (APPS_TOP - APPS_BOTTOM);
end

== matlab function main/MCU Code/Subsystem/cooling_loop_fault_check1 ==
  data: i_avg_long input; cooling_loop_fault output; i_avg_short input
function cooling_loop_fault = fcn(i_avg_long, i_avg_short)
persistent fault;

if isempty(fault)
    fault = 0;
end

i_nom = 0; %Nominal current, A
i_stall = 10; %Stall current, A

if fault == 0
    if i_avg_long > (i_nom+(1-exp(-1))*(i_stall-i_nom))
        fault = 1;
    else
        fault = 0;
    end
else
    if i_avg_short < (i_nom-(1-exp(-1))*(i_nom-i_stall))
        fault = 0;
    else
        fault = 1;
    end
end

cooling_loop_fault = fault;

== matlab function main/MCU Code/MATLAB Function6 ==
  data: ped input; torque output; knob input; TORQUE_MAX input
function torque = fcn(ped, knob, TORQUE_MAX)

t = ped * knob; %knob is 1, constant
torque = min(max(t, 0), 1);

torque = t * TORQUE_MAX;

== matlab function main/MCU Code/MATLAB Function7 ==
  data: driving input; pedal_torque input; direction output; discharge output; enable output; counter output; speed output; speed_mode output; torque output; torque_limit output; motor_speed input
function [direction, discharge, enable, counter, speed, speed_mode, torque, torque_limit]   = fcn(driving, pedal_torque, motor_speed)

persistent my_counter;
if isempty(my_counter)
    my_counter = 0;
else
    my_counter = mod(my_counter + 1, 16);
end

counter = my_counter;

if motor_speed < 500 % rpm, 319rpm = 5kph rules max
    torque_min = 0;
else
    torque_min = -166;
end

torque_max = 166;

if driving == 1
    torque = max(min(pedal_torque, max(0, torque_max)), min(0, torque_min)); %DO NOT TOUCH
    speed = 0;
    direction = 1;
    enable = 1;
    discharge = 0;
    speed_mode = 0;
    torque_limit = 0;
else
    torque = 0;
    speed = 0;
    direction = 1;
    enable = 0;
    discharge = 0;
    speed_mode = 0;
    torque_limit = 0;
end

== matlab function main/MCU Code/MATLAB Function13 ==
  data: pos_raw input; pos output
function pos = fcn(pos_raw)
max_pos = 4096*5; %Min range of servo, SPECIFY
raw = 127.5; %Min range of 8 bit integer

pos = (double(pos_raw)/raw)*(max_pos);

== matlab function main/MCU Code/MATLAB Function9 ==
  data: r_fault_counts output; r_faults output; bpt_sig_mcu input; apps_sig1_mcu input; apps_sig2_mcu input; APPS1_OP input; APPS2_OP input; BPTF_ENGAGED input; APPS1_FAULT input; APPS2_FAULT input; BPTF_FAULT input; r_momentary output
function [r_fault_counts, r_faults, r_momentary] = fcn(bpt_sig_mcu, apps_sig1_mcu, apps_sig2_mcu, APPS1_OP, APPS2_OP, BPTF_ENGAGED, APPS1_FAULT, APPS2_FAULT, BPTF_FAULT)
%#codegen
%To map voltages / integers:
%Pre step down voltages (from sensors, range 0 to 5 V) * 2/3 -> Post step down voltages (0 to 3.3 V, used by mcu)
%Post step down voltages * (4096 / 3.3) -> uint16 (integer) value of variables
%Note: Some values are tweaked after testing to handle noise. 455 -> 435, 0.1 -> 0.13, etc. All values can and should be optimized from testing, especially from testing on the car

%Current operating range (MCU): 0.32 V to 2.67 V
%Brakes considered pressed: 0.40 V
%typical MCU noise: +- 0.03V

persistent fault_counts;
persistent faults;

FAULT_LIMITS = [10, 10, 10, 10, 10, 10, 10, 1];

% initialize persistents
if isempty(fault_counts)
    fault_counts = zeros(1,8);
end

if isempty(faults)
    faults = [false, false, false, false, false, false, false, false];
end

apps1_percent_pressed = (double(apps_sig1_mcu) - APPS1_OP(1))/(APPS1_OP(2) - APPS1_OP(1)); % current travel divided by range of travel
apps2_percent_pressed = (double(apps_sig2_mcu) - APPS2_OP(1))/(APPS2_OP(2) - APPS2_OP(1));

% Clear fault case 8 (two pedals) when apps goes below 5% travel
if (apps1_percent_pressed < 0.05)
    faults(8) = 0;
    fault_counts(8) = 0;
end

% Cases 1-6: APPS or BPT out of operating range (sensor failure)
out_of_bounds = [apps_sig1_mcu < APPS1_FAULT(1), apps_sig1_mcu > APPS1_FAULT(2), ...
                 apps_sig2_mcu < APPS2_FAULT(1), apps_sig2_mcu > APPS2_FAULT(2), ... WHEN APPS DONE PUT BACK
                 bpt_sig_mcu   < BPTF_FAULT(1),  bpt_sig_mcu   > BPTF_FAULT(2)];
% Case 7: Both APPS sensors differ by more than 10% for more than 100ms. 
apps_disagree = abs(apps1_percent_pressed - apps2_percent_pressed) > 0.1;
% Case 8: If APPS is more than 25% pressed and brakes are pressed.
two_pedal = (apps1_percent_pressed >= 0.25) && (bpt_sig_mcu >= BPTF_ENGAGED);

conditions = [out_of_bounds, apps_disagree, two_pedal];

r_momentary = conditions;

conditions(8) = conditions(8) || faults(8); % Case 8 is sticky

% if condition is met but haven't yet triggered fault, increment fault_count.
% if condition is met but already in fault, leave fault_count the same (to
% prevent overflow)
% if condition is not met, zero the count
fault_counts = conditions .* (fault_counts + not(faults));
faults = fault_counts >= FAULT_LIMITS;

r_fault_counts = fault_counts;
r_faults = faults;

== matlab function main/MCU Code/Kalman Filter/MATLAB Function8 ==
  data: v_fl input; v_front output; v_fr input
function v_front = fcn(v_fl,v_fr)

if(v_fl == 0)
    v_front = v_fr;
elseif(v_fr == 0)
    v_front = v_fl;
else
    v_front= (v_fl+v_fr)/2;
end
end

== matlab function main/MCU Code/Kalman Filter/Slip Ratio Calculation1/MATLAB Function ==
  data: fwd_speed input; y output; v_rear input
function y = fcn(fwd_speed,v_rear)

y = (v_rear - fwd_speed)/(max([fwd_speed,0.1]));

== matlab function main/MCU Code/MATLAB Function8 ==
  data: green output; bms input; red output; imd input; t input
function [green,red] = fcn(bms,imd,t)

persistent faulted;

if isempty(faulted)
    faulted=0;
end

if t<4.5
    faulted = 0;
else
    if ~bms || ~imd
        faulted=1;
    end
end

if faulted
    red = 1;
    green = 0;
else
    red = 0;
    green = 1;
end

== matlab function main/MCU Code/Motec Screen/MATLAB Function10 ==
  data: screen_button input; page output
function page = fcn(screen_button)
max_page = 3;
persistent m_page;
if isempty(m_page)
    m_page = 0;
end

if(screen_button~=0)
    if(m_page < max_page)
        m_page=m_page+1;
    else
        m_page = 0;
    end
end

page = m_page;

== matlab function main/MCU Code/Motec Screen/MATLAB Function ==
  data: TC_Button input; TC_switch output
function TC_switch = fcn(TC_Button)
%persistent button;
%if isempty(button)
%    button = 0;
%end

%if(TC_Button~=0)
%    if button == 0
%        button = 1;
%    else
%        button = 0;
%    end
%end
%TC_switch = button;
if (TC_Button)
    TC_switch = 1;
else
    TC_switch = 0;
end

== matlab function main/MCU Code/TC Controller/MATLAB Function1 ==
  data: norm_tc input; lights_out output size=[1 5]; tc_cmd input; driver_cmd input
function lights_out = fcn(norm_tc,tc_cmd,driver_cmd)
    if tc_cmd >= driver_cmd
        lights = [0 0 0 0 0];
    else
        if norm_tc > 0.8
            lights = [1 0 0 0 0];
        elseif norm_tc > 0.6
            lights = [1 1 0 0 0];
        elseif norm_tc > 0.4
            lights = [1 1 1 0 0];
        elseif norm_tc > 0.2
            lights = [1 1 1 1 0];
        else
            lights = [1 1 1 1 1];
        end
    end
    lights_out = double(lights);

== matlab function main/MCU Code/MATLAB Function1 ==
  data: cooling_out_1 output; cooling_out_2 output; cooling_out_3 output; on input; off input
function [cooling_out_1,cooling_out_2,cooling_out_3] = fcn(on, off)
 persistent cooling_1 cooling_2 cooling_3 stage timer_count;
    if isempty(cooling_1)
        cooling_1 = 0;
        cooling_2 = 0;
        cooling_3 = 0;
        stage = 0;
        timer_count = 0;
    end
    
    % Sample time is 0.01s, so 500 ticks = 0.5s
    DELAY_TICKS = double(50);
    
    if off == 1
        cooling_1 = 0;
        cooling_2 = 0;
        cooling_3 = 0;
        stage = 0;
        timer_count = double(0);
    elseif on == 1 && stage == 0
        cooling_1 = 1;
        stage = 1;
        timer_count = double(0);
    end
    
    if stage == 1
        timer_count = timer_count + double(1);
        if timer_count >= DELAY_TICKS
            cooling_2 = 1;
            stage = 2;
            timer_count = double(0);
        end
    elseif stage == 2
        timer_count = timer_count + double(1);
        if timer_count >= DELAY_TICKS
            cooling_3 = 1;
            stage = 3;
        end
    end
    
    cooling_out_1 = cooling_1;
    cooling_out_2 = cooling_2;
    cooling_out_3 = cooling_3;

== matlab function main/MCU Code/TC Controller/Subsystem/Subsystem/MATLAB Function ==
  data: FZ_value input; k_table output; index input; mu_table output; k_opt_lut parameter; mu_opt_lut parameter
function [k_table,mu_table] = fcn(FZ_value, index, k_opt_lut, mu_opt_lut)
    k_table = k_opt_lut(:,:,index); 
    mu_table = mu_opt_lut(:,:,index);
